simulink model "mSubsystem"  (R2023b)
settings: Solver=VariableStepAuto  StartTime=0.0  StopTime=10.0  RelTol=1e-3
settings Model: Creator=uditpant  LastModifiedBy=uditpant

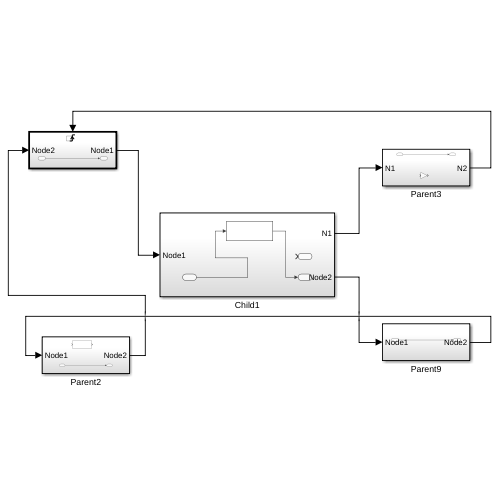
[thumbnail: Simulink's stored preview of the top-level diagram]
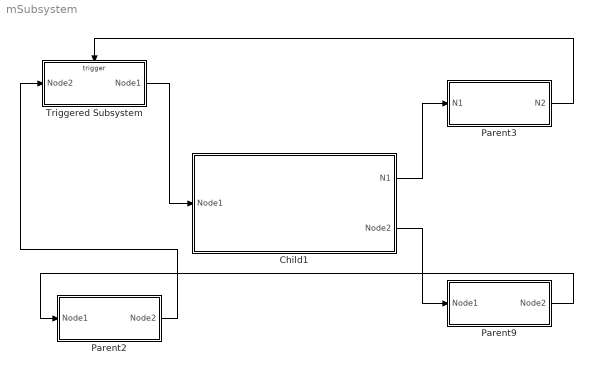
== system mSubsystem ==
  Child1 : Subsystem
  Parent2 : Subsystem
  Parent3 : Subsystem
  Parent9 : Subsystem
  Triggered Subsystem : Subsystem  TreatAsAtomicUnit=on
  wires:
  Triggered Subsystem/1(Node1) -> Child1/1(Node1)
  Parent2/1(Node2) -> Triggered Subsystem/1(Node2)
  Child1/2(Node2) -> Parent9/1(Node1)
  Parent3/1(N2) -> Triggered Subsystem/Trigger
  Parent9/1(Node2) -> Parent2/1(Node1)
  Child1/1(N1) -> Parent3/1(N1)

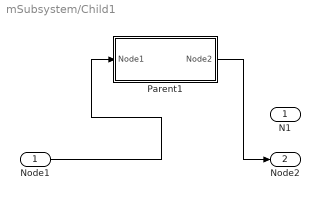
== system mSubsystem/Child1 ==
  Node1 : Inport
  Parent1 : Subsystem
  N1 : Outport
  Node2 : Outport  Port=2
  wires:
  Node1/1 -> Parent1/1(Node1)
  Parent1/1(Node2) -> Node2/1

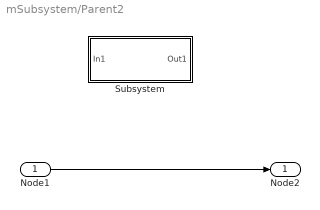
== system mSubsystem/Parent2 ==
  Node1 : Inport
  Subsystem : Subsystem
  Node2 : Outport
  wires:
  Node1/1 -> Node2/1

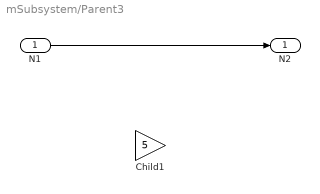
== system mSubsystem/Parent3 ==
  N1 : Inport
  Child1 : Gain  Gain=5
  N2 : Outport
  wires:
  N1/1 -> N2/1

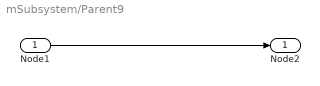
== system mSubsystem/Parent9 ==
  Node1 : Inport
  Node2 : Outport
  wires:
  Node1/1 -> Node2/1

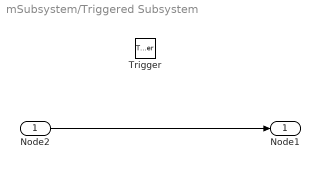
== system mSubsystem/Triggered Subsystem ==
  Node2 : Inport
  Trigger : TriggerPort  VariantControl=(inherit)
  Node1 : Outport
  wires:
  Node2/1 -> Node1/1

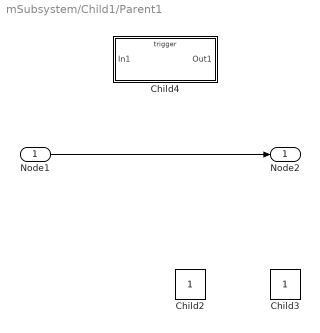
== system mSubsystem/Child1/Parent1 ==
  Node1 : Inport
  Child2 : Constant
  Child3 : Constant
  Child4 : Subsystem  TreatAsAtomicUnit=on
  Node2 : Outport
  wires:
  Node1/1 -> Node2/1

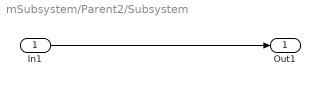
== system mSubsystem/Parent2/Subsystem ==
  In1 : Inport
  Out1 : Outport
  wires:
  In1/1 -> Out1/1

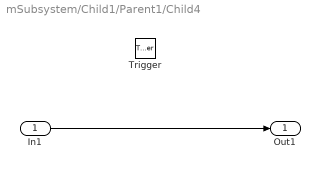
== system mSubsystem/Child1/Parent1/Child4 ==
  In1 : Inport
  Trigger : TriggerPort  VariantControl=(inherit)
  Out1 : Outport
  wires:
  In1/1 -> Out1/1
